simulink model "buscreator_test"  (Simulink 8.4)
settings: Solver=VariableStepDiscrete  StartTime=0.0  StopTime=0  MaxStep=1  RelTol=1e-3
settings Model: Creator=arnaud  LastModifiedBy=arnaud
settings DataIOCC: SaveFormat=Structure  SignalLoggingSaveFormat=Dataset
settings OptimizationCC: ExpressionDepthLimit=128
settings DebuggingCC: UnderspecifiedInitializationDetection=Simplified  MergeDetectMultiDrivingBlocksExec=error  FcnCallInpInsideContextMsg=EnableAllAsError  StateNameClashWarn=none
settings GRTTargetCC: CombineOutputUpdateFcns=on  GRTInterface=off

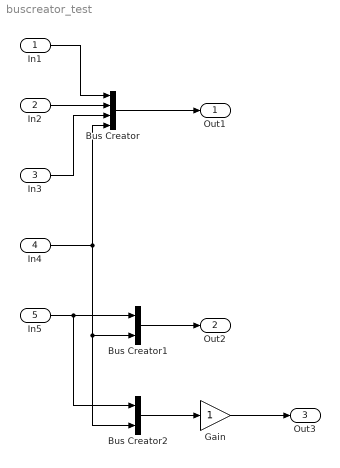
== system buscreator_test ==
  In1 : Inport  OutDataTypeStr=double  PortDimensions=3
  In2 : Inport  Port=2  OutDataTypeStr=int16  PortDimensions=[2 3]  BusOutputAsStruct=on
  In3 : Inport  Port=3  OutDataTypeStr=boolean  PortDimensions=1  BusOutputAsStruct=on
  In4 : Inport  Port=4  OutDataTypeStr=double  PortDimensions=3
  In5 : Inport  Port=5  OutDataTypeStr=double  PortDimensions=1  BusOutputAsStruct=on
  Bus Creator : BusCreator  OutDataTypeStr=Bus: BusA  NonVirtualBus=on
      settings: InheritFromInputs=off
  Bus Creator1 : BusCreator  Inputs=2  OutDataTypeStr=Bus: BusUnif  NonVirtualBus=on
      settings: InheritFromInputs=off
  Bus Creator2 : BusCreator  Inputs=2  OutDataTypeStr=Bus: BusUnif
      settings: InheritFromInputs=off
  Gain : Gain
  Out1 : Outport
  Out2 : Outport  Port=2
  Out3 : Outport  Port=3
  wires:
  In2/1 -> Bus Creator/2
  In1/1 -> Bus Creator/1
  In3/1 -> Bus Creator/3
  Bus Creator/1 -> Out1/1
  Bus Creator1/1 -> Out2/1
  In4/1 -> Bus Creator2/2, Bus Creator1/2, Bus Creator/4
  Bus Creator2/1 -> Gain/1
  In5/1 -> Bus Creator2/1, Bus Creator1/1
  Gain/1 -> Out3/1
